simulink model "qubetemplate_kalman_and_LQR"  (R2021a)
settings: Solver=ode1  StartTime=0.0  StopTime=Tsim  RelTol=1e-3  EnableMultiTasking=on
values from neighbouring files (symbols this model uses):
  h = t(2)-t(1)    [entire_sys_parameter_estimation_grey_box.m]    (also in main.m = 0.02; only_pen_parameter_estimation_grey_box.m; only_pen_parameter_estimation_nonlin_grey_box.m; parameter_estimation_grey_box.m)
  x0 = [pi/4, 0, 0, 0]    [EulerLagrange_script.m]
undefined symbols (not defined in the file or in its folder): Ad, Bd, Cd, Humusoft, K_lqr, Kd, MF634, theta_offset
libraries: sldrtlib x2
settings Model: Creator=rbabuska  LastModifiedBy=chvan
settings SolverCC: AlgebraicLoopSolver=TrustRegion
settings DataIOCC: ExternalInput=ds  LimitDataPoints=on  LoadExternalInput=on  SaveFormat=Array  SignalLoggingSaveFormat=ModelDataLogs  ReturnWorkspaceOutputs=off
settings OptimizationCC: ExpressionDepthLimit=2147483647  LifeSpan=inf
settings DebuggingCC: UnderspecifiedInitializationDetection=Classic  MergeDetectMultiDrivingBlocksExec=none  FcnCallInpInsideContextMsg=warning  StateNameClashWarn=warning  SFUnexpectedBacktrackingDiag=warning  SFNoUnconditionalDefaultTransitionDiag=warning  SFExecutionAtInitializationDiag=none  SFMachineParentedDataDiag=warning  ArithmeticOperatorsInVariantConditions=warning
settings HardwareCC: ProdBitPerPointer=32  ProdBitPerSizeT=32  ProdBitPerPtrDiffT=32  ProdLargestAtomicFloat=None  ProdIntDivRoundTo=Undefined  ProdEndianess=Unspecified  ProdWordSize=32  ProdHWDeviceType=32-bit Generic
settings ModelReferenceCC: PropagateSignalLabelsOutOfModel=off
settings SFSimCC: SimUseLocalCustomCode=off  CustomCodeUndefinedFunction=UseInterfaceOnly
settings RTWCC: RTWUseLocalCustomCode=off
settings CodeAppCC: StateflowObjectComments=on
settings GRTTargetCC: TargetLangStandard=C89/C90 (ANSI)  CombineOutputUpdateFcns=off  GRTInterface=on
settings ConfigComp: CovMetricSettings=dw  CovSaveCumulativeToWorkspaceVar=on  CovSaveSingleToWorkspaceVar=on  CovExternalEMLEnable=off  CovSFcnEnable=off

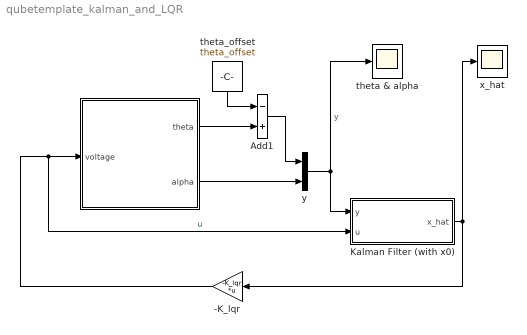
== system qubetemplate_kalman_and_LQR ==
  " " : Subsystem  LoadFcn=hwinit  InitFcn=hwinit  mask{h=h}
      mask prompts: h "Sampling period [s]"
      mask Display:
      | disp('Qube-Servo')
      | port_label('output',1,'theta')
      | port_label('output',2,'alpha')
      | port_label('input',1,'V')
  -K_lqr : Gain  Gain=-K_lqr  Multiplication=Matrix(K*u)
  Add1 : Sum  Inputs=-+
  Kalman Filter (with x0) : Subsystem
  theta & alpha : Scope
  theta_offset : Constant  Value=theta_offset
  x_hat : Scope
  y : Concatenate
  wires:
  -K_lqr/1 -> Kalman Filter (with x0)/2(u), " "/1(voltage)  "u"
  " "/2(alpha) -> y/2
  y/1 -> theta & alpha/1, Kalman Filter (with x0)/1(y)  "y"
  Kalman Filter (with x0)/1(x_hat) -> -K_lqr/1, x_hat/1
  " "/1(theta) -> Add1/2
  Add1/1 -> y/1
  theta_offset/1 -> Add1/1

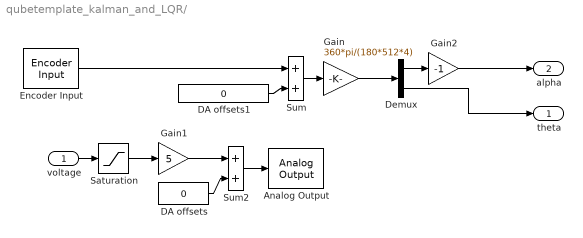
== system qubetemplate_kalman_and_LQR/  ==
  voltage : Inport
  Analog Output : sldrtlib/Analog Output  SampleTime=h  MaxMissedTicks=100  ShowMissedTicks=off  YieldWhenWaiting=off  DrvName=Humusoft/MF634  DrvAddress=4294967295  DrvOptions=0  Channels=[1]  RangeMode=2  VoltRange=1  InitialValue=0  FinalValue=0
      settings: AttributesFormatString=Humusoft\nMF634 [auto]
  DA offsets : Constant  Value=0
  DA offsets1 : Constant  Value=0  SampleTime=h
  Demux : Demux  Outputs=2
  Encoder Input : sldrtlib/Encoder Input  SampleTime=h  MaxMissedTicks=100  ShowMissedTicks=off  YieldWhenWaiting=off  DrvName=Humusoft/MF634  DrvAddress=4294967295  DrvOptions=0  Channels=[1,2]  QuadMode=3  IndexPulse=1  InputFilter=Inf  DataType=1
      settings: AttributesFormatString=Humusoft\nMF634 [auto]
  Gain : Gain  Gain=360*pi/(180*512*4)  SaturateOnIntegerOverflow=on  OutDataTypeStr=Inherit: Same as input  ParamDataTypeStr=Inherit: Same as input
  Gain1 : Gain  Gain=5  SaturateOnIntegerOverflow=on  OutDataTypeStr=Inherit: Same as input  ParamDataTypeStr=Inherit: Same as input
  Gain2 : Gain  Gain=-1  SaturateOnIntegerOverflow=on  OutDataTypeStr=Inherit: Same as input  ParamDataTypeStr=Inherit: Same as input
  Saturation : Saturate  UpperLimit=1  LowerLimit=-1
  Sum : Sum  InputSameDT=on  SaturateOnIntegerOverflow=on  OutDataTypeStr=Inherit: Same as first input
  Sum2 : Sum  InputSameDT=on  SaturateOnIntegerOverflow=on  OutDataTypeStr=Inherit: Same as first input
  theta : Outport  Tag=Cable length
  alpha : Outport  Tag=Cable length  Port=2
  wires:
  Sum/1 -> Gain/1
  DA offsets1/1 -> Sum/2
  Gain1/1 -> Sum2/1
  Sum2/1 -> Analog Output/1
  DA offsets/1 -> Sum2/2
  voltage/1 -> Saturation/1
  Encoder Input/1 -> Sum/1
  Saturation/1 -> Gain1/1
  Demux/1 -> Gain2/1
  Gain/1 -> Demux/1
  Gain2/1 -> alpha/1
  Demux/2 -> theta/1

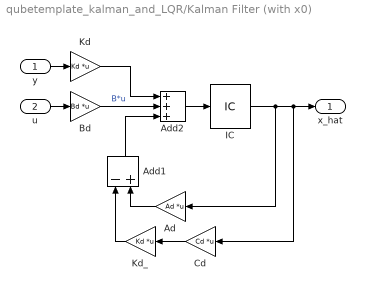
== system qubetemplate_kalman_and_LQR/Kalman Filter (with x0) ==
  y : Inport
  u : Inport  Port=2
  Ad : Gain  Gain=Ad  Multiplication=Matrix(K*u)
  Add1 : Sum  Inputs=-+
  Add2 : Sum  Inputs=+++
  Bd : Gain  Gain=Bd  Multiplication=Matrix(K*u)
  Cd : Gain  Gain=Cd  Multiplication=Matrix(K*u)
  IC : InitialCondition  Value=x0
  Kd : Gain  Gain=Kd  Multiplication=Matrix(K*u)
  Kd_ : Gain  Gain=Kd  Multiplication=Matrix(K*u)
  x_hat : Outport
  wires:
  Add1/1 -> Add2/3
  Ad/1 -> Add1/2
  Bd/1 -> Add2/2  "B*u"
  Kd_/1 -> Add1/1
  Kd/1 -> Add2/1
  Cd/1 -> Kd_/1
  y/1 -> Kd/1
  u/1 -> Bd/1
  IC/1 -> x_hat/1, Cd/1, Ad/1
  Add2/1 -> IC/1
